simulink model "task1model"  (R2025a)
settings: Solver=FixedStepAuto  StartTime=0.0  StopTime=10.0  FixedStep=1e-2  MaxStep=1e-2
model workspace (MAT data in the model file):
  init = [1 1]
settings Model: Creator=hanq  LastModifiedBy=hanq

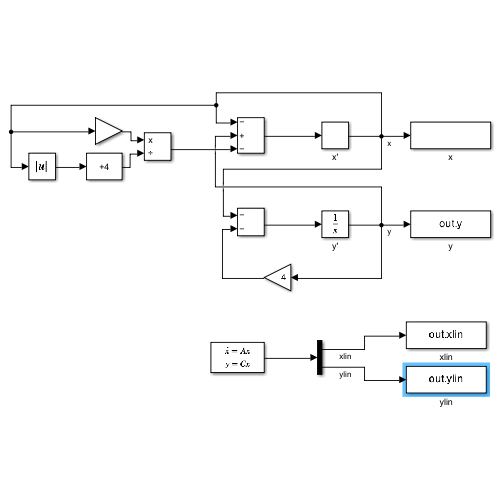
[thumbnail: Simulink's stored preview of the top-level diagram]
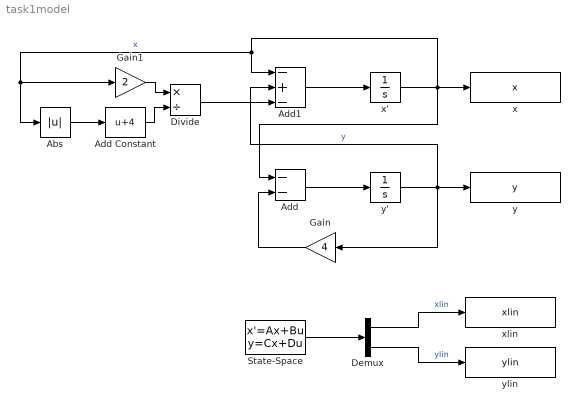
== system task1model ==
  Abs : Abs  SaturateOnIntegerOverflow=off
  Add : Sum  Inputs=--
  Add Constant : Bias  Bias=4  SaturateOnIntegerOverflow=off
  Add1 : Sum  Inputs=-+-
  Demux : Demux  Outputs=2
  Divide : Product  Inputs=*/
  Gain : Gain  Gain=4
  Gain1 : Gain  Gain=2
  State-Space : StateSpace  A=[-3/2,1;-1,-4]  B=zeros(2,0)  C=eye(2)  D=zeros(2,0)  InitialCondition=[1,1]
  x : ToWorkspace  VariableName=x  SaveFormat=Timeseries  SampleTime=-1
  x' : Integrator  InitialCondition=1
  xlin : ToWorkspace  VariableName=xlin  SaveFormat=Timeseries  SampleTime=-1
  y : ToWorkspace  VariableName=y  SaveFormat=Timeseries  SampleTime=-1
  y' : Integrator  InitialCondition=1
  ylin : ToWorkspace  VariableName=ylin  SaveFormat=Timeseries  SampleTime=-1
  wires:
  y'/1 -> Add1/2, y/1, Gain/1  "y"
  x'/1 -> Add1/1, Abs/1, Gain1/1, Add/1, x/1  "x"
  Gain/1 -> Add/2
  Add/1 -> y'/1
  Abs/1 -> Add Constant/1
  Add Constant/1 -> Divide/2
  Gain1/1 -> Divide/1
  Divide/1 -> Add1/3
  Add1/1 -> x'/1
  Demux/1 -> xlin/1  "xlin"
  Demux/2 -> ylin/1  "ylin"
  State-Space/1 -> Demux/1
